simulink model "model1"  (R2021a)
settings: Solver=VariableStepAuto  StartTime=0.0  StopTime=20000  RelTol=1e-3
values from neighbouring files (symbols this model uses):
  A_1 = 20    [skripta.m]
  A_2 = 20    [skripta.m]
  A_c = 250e-4    (= 0.025)    [skripta.m]
  g = 9.81    [skripta.m]
  H_u1 = 4    [skripta.m]
  H_u2 = 4    [skripta.m]
  K_v = 0.5/0.01/60    (= 0.833333333333)    [skripta.m]
settings Model: Creator=Luka  LastModifiedBy=Luka

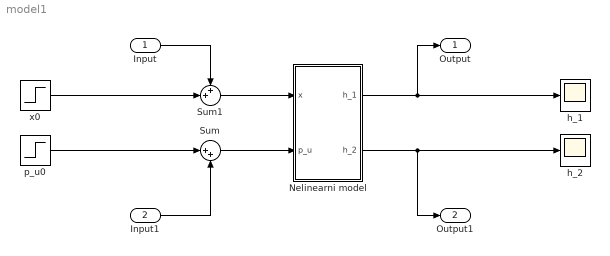
== system model1 ==
  Input : Inport
  Input1 : Inport  Port=2
  Nelinearni model : Subsystem
  Sum : Sum  Inputs=|++
  Sum1 : Sum  Inputs=++|
  h_1 : Scope
  h_2 : Scope
  p_u0 : Step  Time=0  Before=10  After=10  SampleTime=0
  x0 : Step  Time=0  Before=0.05  After=0.05  SampleTime=0
  Output : Outport
  Output1 : Outport  Port=2
  wires:
  Input/1 -> Sum1/1
  x0/1 -> Sum1/2
  p_u0/1 -> Sum/1
  Input1/1 -> Sum/2
  Sum/1 -> Nelinearni model/2(p_u)
  Sum1/1 -> Nelinearni model/1(x)
  Nelinearni model/1(h_1) -> Output/1, h_1/1
  Nelinearni model/2(h_2) -> Output1/1, h_2/1

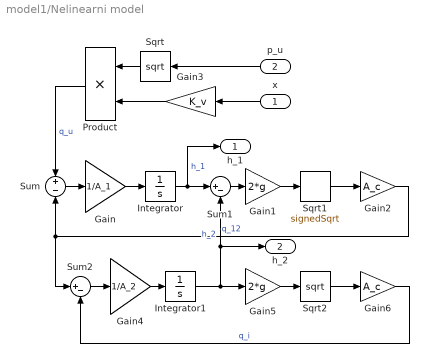
== system model1/Nelinearni model ==
  x : Inport
  p_u : Inport  Port=2
  Gain : Gain  Gain=1/A_1
  Gain1 : Gain  Gain=2*g
  Gain2 : Gain  Gain=A_c
  Gain3 : Gain  Gain=K_v
  Gain4 : Gain  Gain=1/A_2
  Gain5 : Gain  Gain=2*g
  Gain6 : Gain  Gain=A_c
  Integrator : Integrator  InitialCondition=2.831  LimitOutput=on  UpperSaturationLimit=H_u1  LowerSaturationLimit=0
  Integrator1 : Integrator  InitialCondition=1.416  LimitOutput=on  UpperSaturationLimit=H_u2  LowerSaturationLimit=0
  Product : Product
  Sqrt : Sqrt  OutputSignalType=real  SaturateOnIntegerOverflow=on
  Sqrt1 : Sqrt  Operator=signedSqrt  OutputSignalType=real  SaturateOnIntegerOverflow=on
  Sqrt2 : Sqrt  OutputSignalType=real  SaturateOnIntegerOverflow=on
  Sum : Sum  Inputs=+-
  Sum1 : Sum  Inputs=|+-
  Sum2 : Sum  Inputs=|+-
  h_1 : Outport
  h_2 : Outport  Port=2
  wires:
  Gain3/1 -> Product/2
  Sqrt/1 -> Product/1
  Product/1 -> Sum/1  "q_u"
  p_u/1 -> Sqrt/1
  x/1 -> Gain3/1
  Gain2/1 -> Sum2/1, Sum/2  "q_12"
  Sum1/1 -> Gain1/1
  Gain1/1 -> Sqrt1/1
  Sqrt1/1 -> Gain2/1
  Gain6/1 -> Sum2/2  "q_i"
  Gain4/1 -> Integrator1/1
  Gain/1 -> Integrator/1
  Gain5/1 -> Sqrt2/1
  Sqrt2/1 -> Gain6/1
  Sum/1 -> Gain/1
  Integrator/1 -> h_1/1, Sum1/1  "h_1"
  Sum2/1 -> Gain4/1
  Integrator1/1 -> h_2/1, Sum1/2, Gain5/1  "h_2"
